simulink model "battery_system"  (R2022a)
settings: Solver=VariableStepAuto  StartTime=0.0  StopTime=10.0  RelTol=1e-3
values from neighbouring files (symbols this model uses):
  i_user_sim = SIM.i_user_amp    [SimulinkBatterySubsystem_main.m]
  K = diag(diag_vec)    [SimulinkBatterySubsystem_main.m]
  M_cross = V*S_cross*U'    [SimulinkBatterySubsystem_main.m]
  OutputMatrix = SIM.OutputMatrix    [SimulinkBatterySubsystem_main.m]
  SIM = rmfield(SIM,'fsolve_options')    [SimulinkBatterySubsystem_main.m]
  SV_IC = SIM.SV_IC    [SimulinkBatterySubsystem_main.m]
  U_NV_NT = U_null*V_null'    [SimulinkBatterySubsystem_main.m]
undefined symbols (not defined in the file or in its folder): AN, CA, CONS, EL, FLAG, N, P, PROPS, SEP
settings Model: Creator=tyevans  LastModifiedBy=tyevans

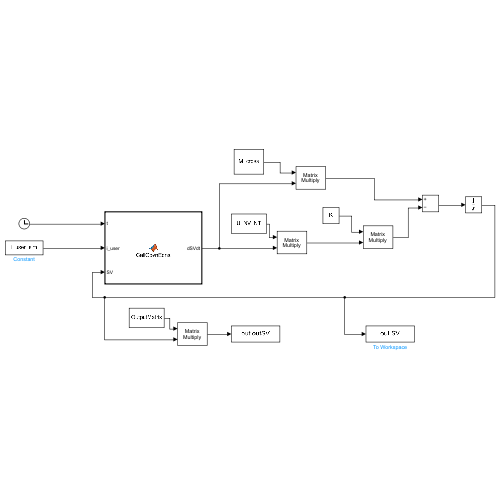
[thumbnail: Simulink's stored preview of the top-level diagram]
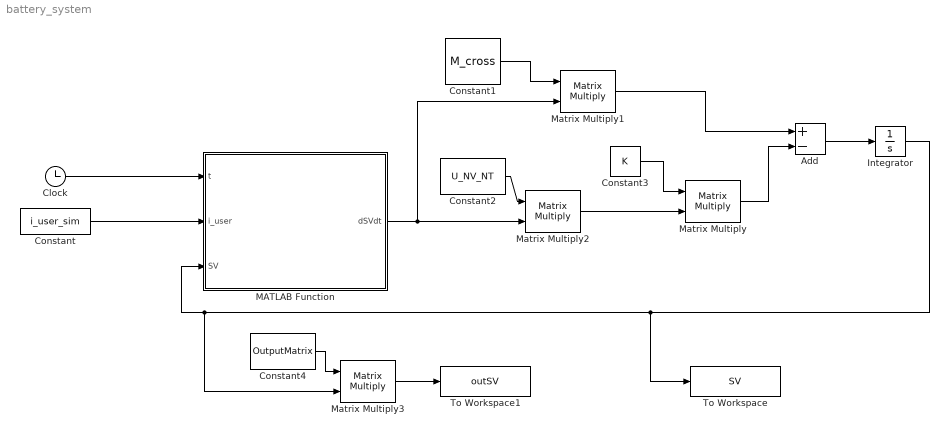
== system battery_system ==
  Add : Sum  Inputs=+-
  Clock : Clock
  Constant : Constant  Value=i_user_sim
  Constant1 : Constant  Value=M_cross  VectorParams1D=off
  Constant2 : Constant  Value=U_NV_NT  VectorParams1D=off
  Constant3 : Constant  Value=K  VectorParams1D=off
  Constant4 : Constant  Value=OutputMatrix  VectorParams1D=off
  Integrator : Integrator  InitialCondition=SV_IC
  MATLAB Function : MATLAB Function  TreatAsAtomicUnit=on
  Matrix Multiply{,1..3} (4 alike) : Product  Multiplication=Matrix(*)
  To Workspace : ToWorkspace  VariableName=SV  SampleTime=-1
  To Workspace1 : ToWorkspace  VariableName=outSV  SampleTime=-1
  wires:
  Constant/1 -> MATLAB Function/2(i_user)
  Clock/1 -> MATLAB Function/1(t)
  MATLAB Function/1(dSVdt) -> Matrix Multiply2/2, Matrix Multiply1/2
  Constant2/1 -> Matrix Multiply2/1
  Constant1/1 -> Matrix Multiply1/1
  Matrix Multiply2/1 -> Matrix Multiply/2
  Constant3/1 -> Matrix Multiply/1
  Matrix Multiply1/1 -> Add/1
  Matrix Multiply/1 -> Add/2
  Add/1 -> Integrator/1
  Integrator/1 -> Matrix Multiply3/2, MATLAB Function/3(SV), To Workspace/1
  Constant4/1 -> Matrix Multiply3/1
  Matrix Multiply3/1 -> To Workspace1/1

== matlab function battery_system/MATLAB Function ==
  data: t input; i_user input; dSVdt output; SV input; AN parameter; CA parameter; SEP parameter; EL parameter; SIM parameter; CONS parameter; P parameter; N parameter; FLAG parameter; PROPS parameter
function dSVdt = CallGovnEqns(t,i_user,SV, AN, CA, SEP, EL, SIM, CONS, P, N, FLAG, PROPS)
% Initialize Output
dSVdt = zeros(N.N_SV_tot,1);

% Call GovnEqns
coder.extrinsic('ConvertStrCallGov')
[dSVdt] = ConvertStrCallGov(t,SV,AN,CA,SEP,EL,SIM,CONS,P,N,FLAG,PROPS,i_user);

end
